simulink model "dq_abc"  (R2019b)
settings: Solver=VariableStepAuto  StartTime=0.0  StopTime=10.0  RelTol=1e-3
libraries: powerlib_meascontrol x1
settings Model: Creator=SASTRA  LastModifiedBy=SASTRA

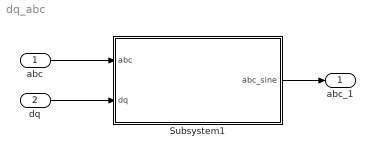
== system dq_abc ==
  abc : Inport
  dq : Inport  Port=2
  Subsystem1 : Subsystem
  abc_1 : Outport
  wires:
  abc/1 -> Subsystem1/1(abc)
  dq/1 -> Subsystem1/2(dq)
  Subsystem1/1(abc_sine) -> abc_1/1

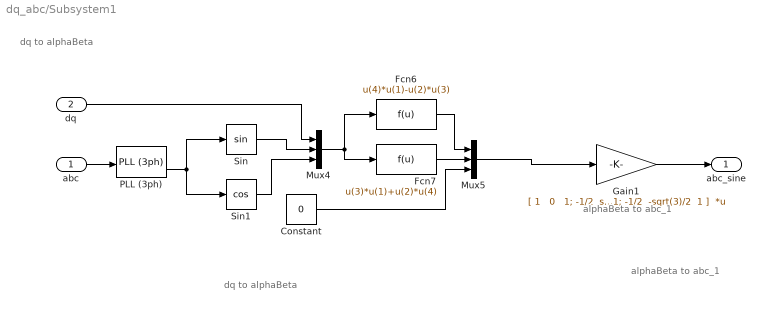
== system dq_abc/Subsystem1 ==
  note: alphaBeta to abc_1
  note: alphaBeta to abc_1
  note: dq to alphaBeta
  note: dq to alphaBeta
  abc : Inport
  dq : Inport  Port=2
  Constant : Constant  Value=0
  Fcn6 : Fcn  Expr=u(4)*u(1)-u(2)*u(3)
  Fcn7 : Fcn  Expr=u(3)*u(1)+u(2)*u(4)
  Gain1 : Gain  Gain="[ 1   0   1; -1/2  sqrt(3)/2   1; -1/2  -sqrt(3)/2  1 ]"  Multiplication=Matrix(K*u) (u vector)
  Mux4 : Mux  Inputs=3
  Mux5 : Mux  Inputs=3
  PLL (3ph) : powerlib_meascontrol/PLL/PLL (3ph)  Fmin=45  Par_Init=[0, 50]  ParK=[180, 3200, 1]  TcD=1e-4  MaxRateChangeFreq=12  FilterCutOffFreq=25  Ts=0  AGC=on
      settings: SourceProductName=Simscape Electrical
  Sin : Trigonometry
  Sin1 : Trigonometry  Operator=cos
  abc_sine : Outport
  wires:
  Mux4/1 -> Fcn6/1, Fcn7/1
  dq/1 -> Mux4/1
  PLL (3ph)/2 -> Sin1/1, Sin/1
  Mux5/1 -> Gain1/1
  Constant/1 -> Mux5/3
  Fcn6/1 -> Mux5/1
  Fcn7/1 -> Mux5/2
  Gain1/1 -> abc_sine/1
  Sin/1 -> Mux4/2
  Sin1/1 -> Mux4/3
  abc/1 -> PLL (3ph)/1
